simulink model "LLC_HalfBridge_Converter"  (R2020a)
settings: Solver=ode23tb  StartTime=0.0  StopTime=0.02  RelTol=1e-7  AbsTol=1e-7
libraries: powerlib x19, powerlib_meascontrol x3, eePowerMeasurement x2
settings Model: Creator=erenb  LastModifiedBy=erenb
settings DataIOCC: ReturnWorkspaceOutputs=off
settings DebuggingCC: ArithmeticOperatorsInVariantConditions=warning
settings SFSimCC: CustomCodeUndefinedFunction=UseInterfaceOnly

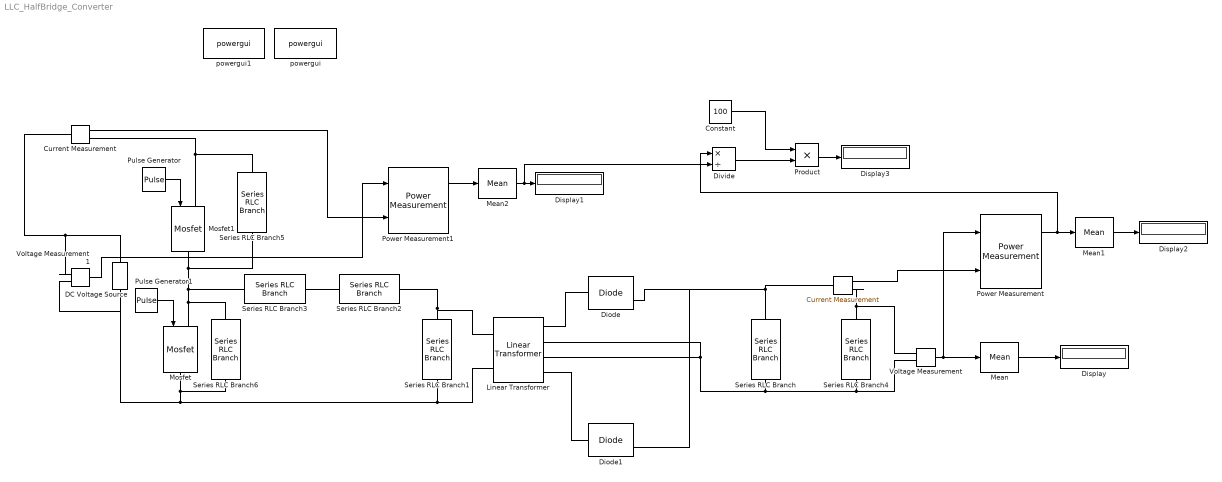
== system LLC_HalfBridge_Converter ==
  " " : powerlib/Measurements/Current Measurement  PhasorSimulation=off  OutputType=Complex  PSBequivalent=0
  Constant : Constant  Value=100
  Current Measurement : powerlib/Measurements/Current Measurement  PhasorSimulation=off  OutputType=Complex  PSBequivalent=0
  DC Voltage Source : powerlib/Electrical Sources/DC Voltage Source  Amplitude=390  Measurements=None
  Diode : powerlib/Power Electronics/Diode  Ron=700e-3  Lon=0  Vf=0.08  IC=0  UseSnubber=0  Rs=inf  Cs=250e-3  Measurements=on
  Diode1 : powerlib/Power Electronics/Diode  Ron=700e-3  Lon=0  Vf=0.08  IC=0  UseSnubber=0  Rs=inf  Cs=250e-3  Measurements=on
  Display{,1..3} (4 alike) : Display
  Divide : Product  Inputs=*/
  Linear Transformer : powerlib/Elements/Linear Transformer  UNITS=pu  NominalPower=[ 300 113685 ]  winding1=[350 0 0]  winding2=[350/6.5 0 0]  ThreeWindings=on  winding3=[350/6.5 0 0]  RmLm=[100.02 100]  Measurements=None  DataType=off
  Mean : powerlib_meascontrol/Measurements/Mean  Freq=110000  Vinit=0  Ts=5e-8
  Mean1 : powerlib_meascontrol/Measurements/Mean  Freq=110000  Vinit=0  Ts=5e-8
  Mean2 : powerlib_meascontrol/Measurements/Mean  Freq=110000  Vinit=0  Ts=5e-8
  Mosfet : powerlib/Power Electronics/Mosfet  Ron=0.001  Lon=0  Rd=0.001  Vfd=0  IC=0  Rs=1e5  Cs=1e-6  Measurements=off
  Mosfet1 : powerlib/Power Electronics/Mosfet  Ron=0.001  Lon=0  Rd=0.001  Vfd=0  IC=0  Rs=1e5  Cs=1e-6  Measurements=off
  Power Measurement : eePowerMeasurement/Power Measurement  LabelModeActiveChoice=Discrete  F=113685  K=[0]  Ts=1/113685
      settings: SourceProductBaseCode=PS
  Power Measurement1 : eePowerMeasurement/Power Measurement  LabelModeActiveChoice=Discrete  F=113685  K=[0]  Ts=1/113685
      settings: SourceProductBaseCode=PS
  Product : Product
  Pulse Generator : DiscretePulseGenerator  PulseType=Time based  Amplitude=390  Period=1/113685  PulseWidth=50  PhaseDelay=1e-6
  Pulse Generator1 : DiscretePulseGenerator  PulseType=Time based  Amplitude=390  Period=1/113685  PulseWidth=50  PhaseDelay=5e-6
  Series RLC Branch : powerlib/Elements/Series RLC Branch  LConnTagsString=__new0  RConnTagsString=__new0  BranchType=C  Resistance=1  Inductance=1e-3  SetiL0=off  InitialCurrent=0  Capacitance=1000e-6  Setx0=off  InitialVoltage=0  Measurements=None
  Series RLC Branch1 : powerlib/Elements/Series RLC Branch  LConnTagsString=__new0  RConnTagsString=__new0  BranchType=L  Resistance=1  Inductance=500e-6  SetiL0=off  InitialCurrent=0  Capacitance=1e-6  Setx0=off  InitialVoltage=0  Measurements=None
  Series RLC Branch2 : powerlib/Elements/Series RLC Branch  LConnTagsString=__new0  RConnTagsString=__new0  BranchType=L  Resistance=1  Inductance=50e-6  SetiL0=off  InitialCurrent=0  Capacitance=1e-6  Setx0=off  InitialVoltage=0  Measurements=None
  Series RLC Branch3 : powerlib/Elements/Series RLC Branch  LConnTagsString=__new0  RConnTagsString=__new0  BranchType=C  Resistance=1  Inductance=1e-3  SetiL0=off  InitialCurrent=0  Capacitance=14e-9  Setx0=off  InitialVoltage=0  Measurements=None
  Series RLC Branch4 : powerlib/Elements/Series RLC Branch  LConnTagsString=__new0  RConnTagsString=__new0  BranchType=R  Resistance=7.155  Inductance=1e-3  SetiL0=off  InitialCurrent=0  Capacitance=1e-6  Setx0=off  InitialVoltage=0  Measurements=None
  Series RLC Branch5 : powerlib/Elements/Series RLC Branch  LConnTagsString=__new0  RConnTagsString=__new0  BranchType=RC  Resistance=580  Inductance=1e-3  SetiL0=off  InitialCurrent=0  Capacitance=100e-3  Setx0=off  InitialVoltage=0  Measurements=None
  Series RLC Branch6 : powerlib/Elements/Series RLC Branch  LConnTagsString=__new0  RConnTagsString=__new0  BranchType=RC  Resistance=580  Inductance=1e-3  SetiL0=off  InitialCurrent=0  Capacitance=100e-3  Setx0=off  InitialVoltage=0  Measurements=None
  Voltage Measurement : powerlib/Measurements/Voltage Measurement  PhasorSimulation=off  OutputType=Complex  PSBequivalent=0
  Voltage Measurement1 : powerlib/Measurements/Voltage Measurement  PhasorSimulation=off  OutputType=Complex  PSBequivalent=0
  powergui : powerlib/powergui  Priority=1  SimulationMode=Discrete  SampleTime=5e-8  frequency=60  Iterations=50  frequencyindice=0  Pbase=100e6  ErrMax=1e-4  UnitsV=kV  UnitsW=MW  buscounter=0  FunctionMessages=on  echomessages=off  EnableUseOfTLC=off  CurrentSourceSwitches=off  DisableSnubberDevices=off  DisableRonSwitches=off  DisableVfSwitches=off  DisplayEquations=off  AutomaticDiscreteSolvers=off  SolverType=Tustin/Backward Euler (TBE)  Interpol=off  ExternalGateDelay=off  methode=off  Ts=100  x0status=blocks  SPID=on  SwTol=0  HookPort=off  NonlinearTolerance=1e-4  nMaxIteration=100  ContinueOnMaxIteration=off  RestoreLinks=warning  ResistiveCurrentMeasurement=off  Frange=[0:2:500]  Ylog=off  Xlog=on  ShowGrid=off  save=off  variable=ZData  structure=0  ZoomFFT=off  StartTime=0.0  cycles=1  DisplayStyle=1  fundamental=60  FreqAxis=off  MaxFrequency=1000  frequencyindicesteady=1  RmsSteady=1  display=off
  powergui1 : powerlib/powergui  Priority=1  SimulationMode=Continuous  SampleTime=50e-6  frequency=60  Iterations=50  frequencyindice=60  Pbase=100e6  ErrMax=1e-4  UnitsV=kV  UnitsW=MW  buscounter=0  FunctionMessages=off  echomessages=off  EnableUseOfTLC=off  CurrentSourceSwitches=off  DisableSnubberDevices=off  DisableRonSwitches=off  DisableVfSwitches=off  DisplayEquations=off  AutomaticDiscreteSolvers=off  SolverType=Tustin/Backward Euler (TBE)  Interpol=off  ExternalGateDelay=off  methode=off  Ts=100  x0status=blocks  SPID=on  SwTol=0  HookPort=off  NonlinearTolerance=1e-4  nMaxIteration=100  ContinueOnMaxIteration=off  RestoreLinks=warning  ResistiveCurrentMeasurement=off  Frange=[0:2:500]  Ylog=off  Xlog=on  ShowGrid=off  save=off  variable=ZData  structure=0  ZoomFFT=off  StartTime=0.0  cycles=1  DisplayStyle=1  fundamental=60  FreqAxis=off  MaxFrequency=1000  frequencyindicesteady=1  RmsSteady=1  display=off
  wires:
  Pulse Generator1/1 -> Mosfet/1
  Pulse Generator/1 -> Mosfet1/1
  Voltage Measurement/1 -> Mean/1, Power Measurement/1
  Mean/1 -> Display/1
  " "/1 -> Power Measurement/2
  Current Measurement/1 -> Power Measurement1/2
  Voltage Measurement1/1 -> Power Measurement1/1
  Mean1/1 -> Display2/1
  Power Measurement/1 -> Divide/1, Mean1/1
  Power Measurement1/1 -> Mean2/1
  Mean2/1 -> Divide/2, Display1/1
  Divide/1 -> Product/2
  Constant/1 -> Product/1
  Product/1 -> Display3/1
  connections:
  Series RLC Branch1/RConn1 -- Linear Transformer/LConn2 -- Voltage Measurement1/LConn2 -- DC Voltage Source/LConn1 -- Mosfet/RConn1 -- Series RLC Branch6/RConn1
  Series RLC Branch2/RConn1 -- Linear Transformer/LConn1 -- Series RLC Branch1/LConn1
  Diode1/RConn1 -- Diode/RConn1 -- Series RLC Branch/LConn1 -- " "/LConn1
  Series RLC Branch3/RConn1 -- Series RLC Branch2/LConn1
  Mosfet1/LConn1 -- Series RLC Branch5/LConn1 -- Current Measurement/RConn1
  Mosfet/LConn1 -- Series RLC Branch6/LConn1 -- Series RLC Branch5/RConn1 -- Mosfet1/RConn1 -- Series RLC Branch3/LConn1
  Diode/LConn1 -- Linear Transformer/RConn1
  Series RLC Branch/RConn1 -- Voltage Measurement/LConn2 -- Series RLC Branch4/RConn1 -- Linear Transformer/RConn2 -- Linear Transformer/RConn3
  Diode1/LConn1 -- Linear Transformer/RConn4
  " "/RConn1 -- Voltage Measurement/LConn1 -- Series RLC Branch4/LConn1
  Current Measurement/LConn1 -- Voltage Measurement1/LConn1 -- DC Voltage Source/RConn1
